simulink model "ch7example3"  (Simulink 5.0)
settings: Solver=FixedStepDiscrete  StartTime=0.0  StopTime=10.0  FixedStep=1/10  RelTol=1e-3
libraries: commrandsrc2 x1
settings Model: LastModifiedBy=shaoyubin

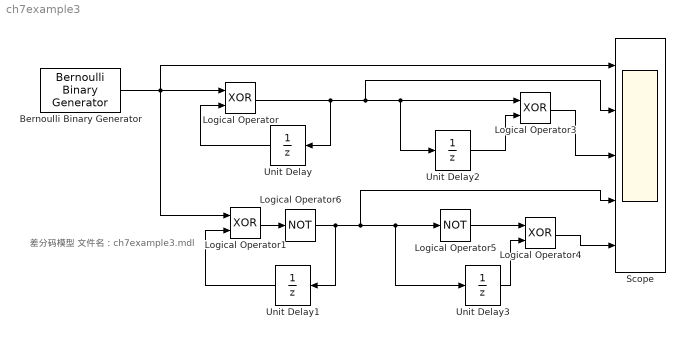
== system ch7example3 ==
  note: 差分码模型
      | 文件名：ch7example3.mdl
  Bernoulli Binary Generator : commrandsrc2/Bernoulli Binary Generator  P=0.5  seed=61  Ts=1  frameBased=off  sampPerFrame=1  orient=off
  Logical Operator{,1,3..4} (4 alike) : Logic  Operator=XOR  AllPortsSameDT=off
  Logical Operator5 : Logic  Operator=NOT  AllPortsSameDT=off
  Logical Operator6 : Logic  Operator=NOT  AllPortsSameDT=off
  Scope : Scope  NumInputPorts=5
      settings: TickLabels=off  YMin=-2~-2~-2~-2~-2  YMax=2~2~2~2~2
  Unit Delay : UnitDelay  Orientation=left
  Unit Delay1 : UnitDelay  Orientation=left
  Unit Delay2 : UnitDelay
  Unit Delay3 : UnitDelay
  wires:
  Bernoulli Binary Generator/1 -> Logical Operator1/1, Logical Operator/1, Scope/1
  Logical Operator/1 -> Unit Delay/1, Logical Operator3/1, Unit Delay2/1, Scope/2
  Unit Delay/1 -> Logical Operator/2
  Logical Operator1/1 -> Logical Operator6/1
  Unit Delay1/1 -> Logical Operator1/2
  Unit Delay2/1 -> Logical Operator3/2
  Unit Delay3/1 -> Logical Operator4/2
  Logical Operator5/1 -> Logical Operator4/1
  Logical Operator6/1 -> Unit Delay1/1, Unit Delay3/1, Logical Operator5/1, Scope/4
  Logical Operator3/1 -> Scope/3
  Logical Operator4/1 -> Scope/5
